simulink model "pendule_inv_capteur_etu"  (R2021a)
settings: Solver=VariableStepAuto  StartTime=0.0  StopTime=100  RelTol=1e-3
model workspace (MAT data in the model file):
  xpre = Simulink.Parameter
  xpre.Value = Simulink.data.Expression
  xpre.Value.ExpressionString = "x0(1)"
  xpre.DataType = 'auto'
  xpre.Dimensions = -1
values from neighbouring files (symbols this model uses):
  g = 9.81    [simu_pendule_inv_capteur_etu.m]    (also in simu_pendule_inv_echant_etu.m; simu_pendule_inv_etu.m)
  K = [10 1]    [simu_pendule_inv_capteur_etu.m]    (also in simu_pendule_inv_echant_etu.m = [30 10]; simu_pendule_inv_etu.m = [30 10])
  l = 10    [simu_pendule_inv_capteur_etu.m]    (also in simu_pendule_inv_echant_etu.m; simu_pendule_inv_etu.m)
  ue = 0    [simu_pendule_inv_capteur_etu.m]    (also in simu_pendule_inv_echant_etu.m; simu_pendule_inv_etu.m)
  x0 = [pi/20 0]'    [simu_pendule_inv_capteur_etu.m]    (also in simu_pendule_inv_echant_etu.m; simu_pendule_inv_etu.m = [pi/10 0]')
  xe = [0 0]'    [simu_pendule_inv_capteur_etu.m]    (also in simu_pendule_inv_echant_etu.m; simu_pendule_inv_etu.m)
settings Model: Creator=Jed  LastModifiedBy=jmoutahi

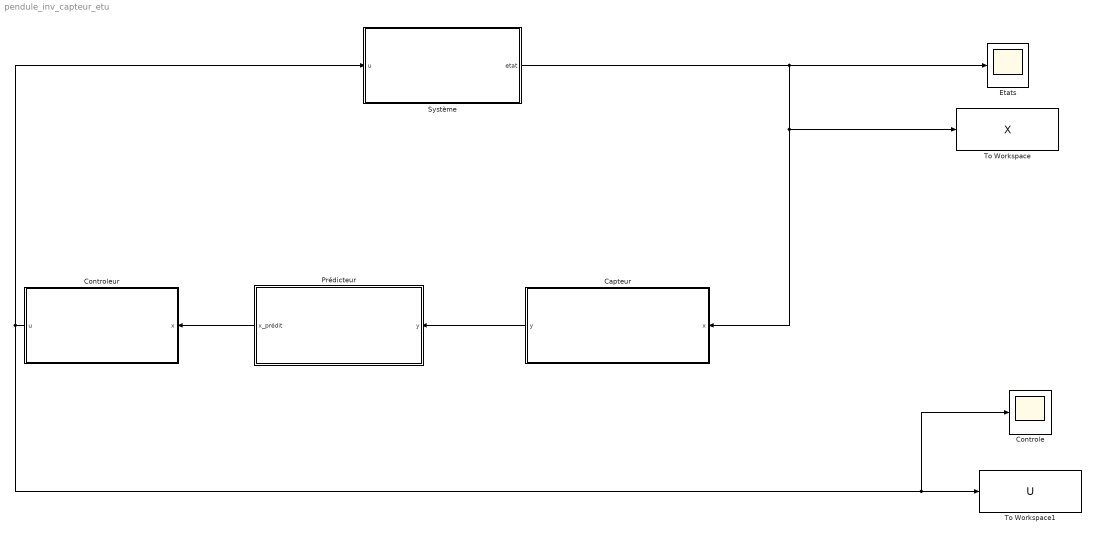
== system pendule_inv_capteur_etu ==
  Capteur : Subsystem
  Controle : Scope
  Controleur : Subsystem
  Etats : Scope
  Prédicteur : Subsystem
  Système : Subsystem
  To Workspace : ToWorkspace  VariableName=X  SaveFormat=Timeseries  SampleTime=-1
  To Workspace1 : ToWorkspace  VariableName=U  SaveFormat=Timeseries  SampleTime=-1
  wires:
  Controleur/1(u) -> Système/1(u), Controle/1, To Workspace1/1
  Système/1(etat) -> To Workspace/1, Capteur/1(x), Etats/1
  Prédicteur/1(x_prédit) -> Controleur/1(x)
  Capteur/1(y) -> Prédicteur/1(y)

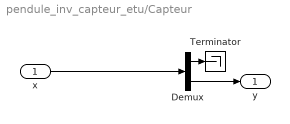
== system pendule_inv_capteur_etu/Capteur ==
  x : Inport
  Demux : Demux  Outputs=2
  Terminator : Terminator
  y : Outport
  wires:
  x/1 -> Demux/1
  Demux/2 -> y/1
  Demux/1 -> Terminator/1

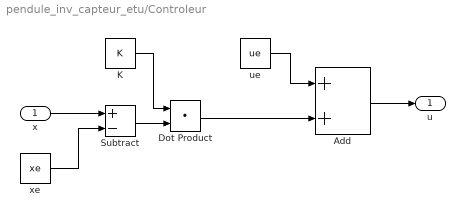
== system pendule_inv_capteur_etu/Controleur ==
  x : Inport
  Add : Sum
  Dot Product : DotProduct  InputSameDT=on  OutDataTypeStr=Inherit: Inherit via internal rule
  K : Constant  Value=K
  Subtract : Sum  Inputs=+-
  ue : Constant  Value=ue
  xe : Constant  Value=xe
  u : Outport
  wires:
  Add/1 -> u/1
  ue/1 -> Add/1
  x/1 -> Subtract/1
  xe/1 -> Subtract/2
  Dot Product/1 -> Add/2
  Subtract/1 -> Dot Product/2
  K/1 -> Dot Product/1

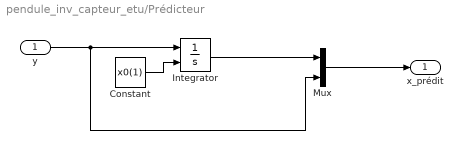
== system pendule_inv_capteur_etu/Prédicteur ==
  y : Inport
  Constant : Constant  Value=x0(1)
  Integrator : Integrator  InitialConditionSource=external
  Mux : Mux  Inputs=2
  x_prédit : Outport
  wires:
  y/1 -> Integrator/1, Mux/2
  Integrator/1 -> Mux/1
  Constant/1 -> Integrator/2
  Mux/1 -> x_prédit/1

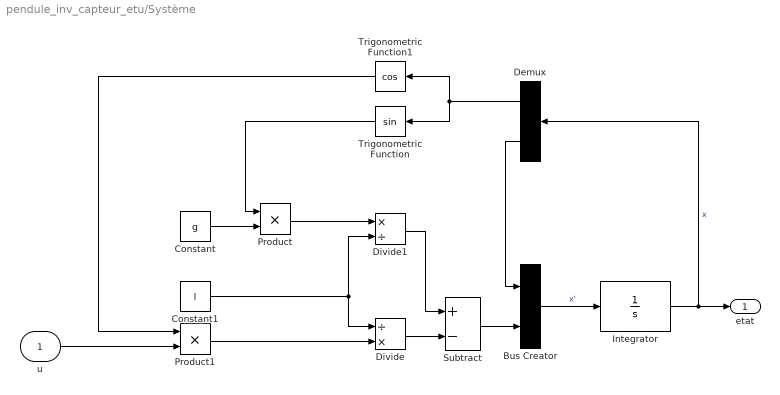
== system pendule_inv_capteur_etu/Système ==
  u : Inport
  Bus Creator : BusCreator  Inputs=2
  Constant : Constant  Value=g
  Constant1 : Constant  Value=l
  Demux : Demux  Outputs=2
  Divide : Product  Inputs=/*
  Divide1 : Product  Inputs=*/
  Integrator : Integrator  InitialCondition=x0
  Product : Product
  Product1 : Product
  Subtract : Sum  Inputs=+-
  Trigonometric Function : Trigonometry
  Trigonometric Function1 : Trigonometry  Operator=cos
  etat : Outport
  wires:
  Integrator/1 -> etat/1, Demux/1  "x"
  Bus Creator/1 -> Integrator/1  "x'"
  Demux/2 -> Bus Creator/1
  Demux/1 -> Trigonometric Function1/1, Trigonometric Function/1
  Subtract/1 -> Bus Creator/2
  u/1 -> Product1/2
  Trigonometric Function1/1 -> Product1/1
  Divide/1 -> Subtract/2
  Constant1/1 -> Divide1/2, Divide/1
  Product1/1 -> Divide/2
  Constant/1 -> Product/2
  Trigonometric Function/1 -> Product/1
  Product/1 -> Divide1/1
  Divide1/1 -> Subtract/1
